simulink subsystem "lqr_position"  (R2025b)
settings: Solver=VariableStepAuto  StartTime=0.0  StopTime=10.0  RelTol=1e-3
values from neighbouring files (symbols this model uses):
  A_trans = [ ... (first row only)    [params.m]
  B_trans = [ ... (first row only)    [params.m]
  C_trans = [ ... (first row only)    [params.m]
  g = 9.81    [params.m]    (also in params_1dof.m; params_3dof.m)
  K_trans = K_erw(1:3, 1:6)    [params.m]
  Ki_trans = K_erw(1:3, 7:9)    [params.m]
  m = 1.210    (= 1.21)    [params.m]    (also in params_1dof.m = 1.014; params_3dof.m = 1.014)
undefined symbols (not defined in the file or in its folder): DiscIntNeverNeededParam
settings Model: Creator=schwmaxi  LastModifiedBy=schwmaxi

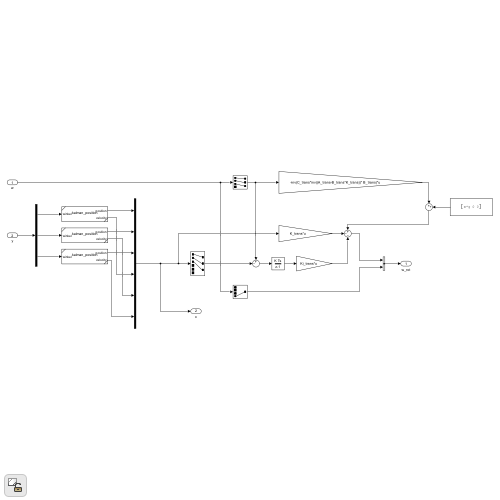
[thumbnail: Simulink's stored preview of the top-level diagram]
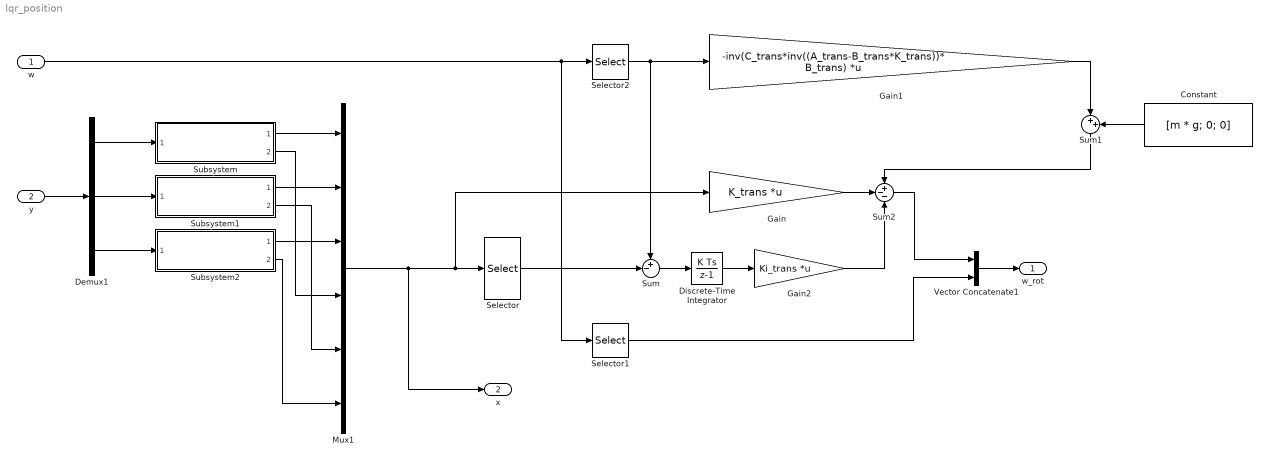
== system lqr_position ==
  w : Inport
  y : Inport  Port=2
  Constant : Constant  Value=[m * g; 0; 0]
  Demux1 : Demux  Outputs=3
  Discrete-Time Integrator : DiscreteIntegrator  SampleTime=-1  ICPrevOutput=DiscIntNeverNeededParam  ICPrevScaledInput=DiscIntNeverNeededParam
  Gain : Gain  Gain=K_trans  Multiplication=Matrix(K*u)
  Gain1 : Gain  Gain=-inv(C_trans*inv((A_trans-B_trans*K_trans))* B_trans)  Multiplication=Matrix(K*u)
  Gain2 : Gain  Gain=Ki_trans  Multiplication=Matrix(K*u)
  Mux1 : Mux  Inputs=6
  Selector : Selector  InputPortWidth=6  IndexOptions=Index vector (dialog)  Indices=[1 2 3]  OutputSizes=1
  Selector1 : Selector  InputPortWidth=4  IndexOptions=Index vector (dialog)  Indices=[4]  OutputSizes=1
  Selector2 : Selector  InputPortWidth=4  IndexOptions=Index vector (dialog)  Indices=[1 2 3]  OutputSizes=1
  Subsystem : Subsystem  ReferencedSubsystem=kalman_position
  Subsystem1 : Subsystem  ReferencedSubsystem=kalman_position
  Subsystem2 : Subsystem  ReferencedSubsystem=kalman_position
  Sum : Sum  Inputs=+-|
  Sum1 : Sum  Inputs=|++
  Sum2 : Sum  Inputs=+--
  Vector Concatenate1 : Concatenate
  w_rot : Outport
  x : Outport  Port=2
  wires:
  Mux1/1 -> Gain/1, Selector/1, x/1
  y/1 -> Demux1/1
  Demux1/1 -> Subsystem/1
  Subsystem/1 -> Mux1/1
  Subsystem/2 -> Mux1/4
  Demux1/2 -> Subsystem1/1
  Subsystem1/1 -> Mux1/2
  Subsystem1/2 -> Mux1/5
  Subsystem2/1 -> Mux1/3
  Demux1/3 -> Subsystem2/1
  Subsystem2/2 -> Mux1/6
  Sum2/1 -> Vector Concatenate1/1
  w/1 -> Selector1/1, Selector2/1
  Vector Concatenate1/1 -> w_rot/1
  Selector2/1 -> Gain1/1, Sum/1
  Selector/1 -> Sum/2
  Gain/1 -> Sum2/2
  Selector1/1 -> Vector Concatenate1/2
  Sum1/1 -> Sum2/1
  Gain2/1 -> Sum2/3
  Constant/1 -> Sum1/2
  Gain1/1 -> Sum1/1
  Discrete-Time Integrator/1 -> Gain2/1
  Sum/1 -> Discrete-Time Integrator/1
